simulink model "px4_allSensorsDemo"  (R2018b)
settings: Solver=FixedStepAuto  StartTime=0.0  StopTime=inf  RelTol=1e-3  EnableMultiTasking=on
libraries: px4Sensorslib x3, simulink_extras x3, px4uORBlib x2
settings Model: SimulationMode=external  ExtModeEnableFloating=off  ExtModeTrigDuration=10  Creator=The MathWorks, Inc.  LastModifiedBy=Tejas Rajopadhye
settings SolverCC: PositivePriorityOrder=on
settings DataIOCC: ReturnWorkspaceOutputs=on
settings OptimizationCC: EnhancedBackFolding=on  PassReuseOutputArgsAs=Individual arguments  MaxStackSize=64  OptimizeBlockOrder=speed  DifferentSizesBufferReuse=on  OptimizationCustomize=off
settings DebuggingCC: ParameterTunabilityLossMsg=error
settings HardwareCC: ProdBitPerPointer=32  ProdBitPerSizeT=32  ProdBitPerPtrDiffT=32  ProdLargestAtomicInteger=Long  ProdLargestAtomicFloat=Double  ProdWordSize=32  ProdLongLongMode=on  ProdHWDeviceType=ARM Compatible->ARM Cortex
settings SFSimCC: MATLABDynamicMemAlloc=off
settings RTWCC: SystemTargetFile=ert.tlc  HardwareBoard=PX4 Pixhawk 4  TLCOptions="-aInlineSetEventsForThisBaseRateFcn=TLC_FALSE -aSuppressMultiTaskScheduler=TLC_FALSE  -aRateBasedStepFcn=0"  TemplateMakefile=ert_default_tmf  GenerateReport=on  Toolchain=GNU Tools for PX4 Autopilots  IncludeHyperlinkInReport=on  LaunchReport=on  TargetLang=C++  GenerateTraceInfo=on  GenerateTraceReport=on  GenerateTraceReportSl=on  GenerateTraceReportSf=on  GenerateTraceReportEml=on
settings CodeAppCC: ForceParamTrailComments=on  IgnoreCustomStorageClasses=off  OperatorAnnotations=on  SimulinkDataObjDesc=on  SFDataObjDesc=on  InsertBlockDesc=on

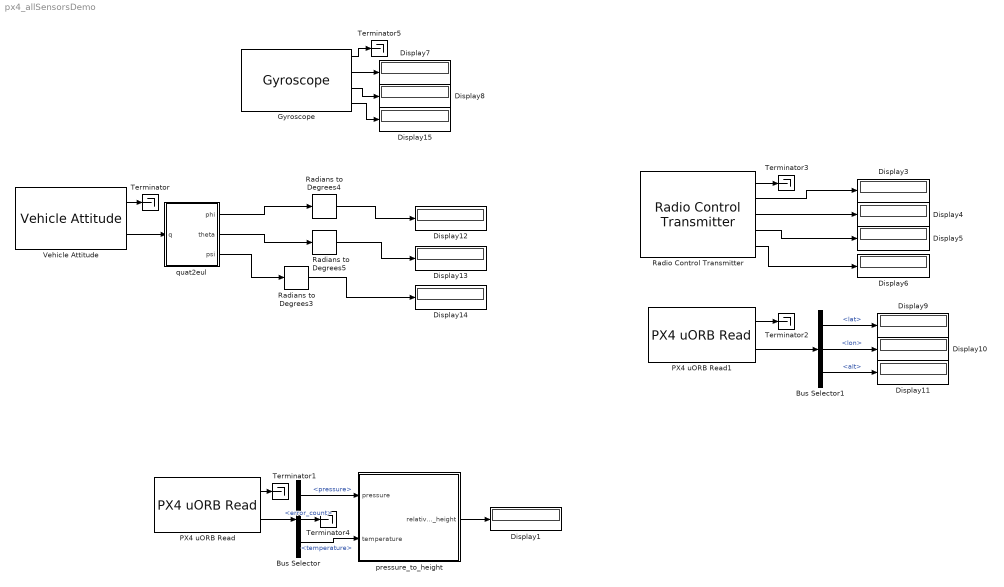
== system px4_allSensorsDemo ==
  Bus Selector : BusSelector  OutputSignals=pressure,error_count,temperature
  Bus Selector1 : BusSelector  OutputSignals=lat,lon,alt
  Display{1,3..15} (14 alike) : Display
  Gyroscope : px4Sensorslib/Gyroscope  uorbTimeStamp=off  BlockingMode=off  BlockTimeout=1e-3  sampleTime=1/250
      settings: SourceProductName=Embedded Coder Support Package for PX4 Autopilots
  PX4 uORB Read : px4uORBlib/PX4 uORB Read  uORBTopic=sensor_baro  sampleTime=-1  BlockingMode=off  BlockTimeout=1e-3
      settings: SourceProductName=Embedded Coder Support Package for PX4 Autopilots
  PX4 uORB Read1 : px4uORBlib/PX4 uORB Read  uORBTopic=vehicle_gps_position  sampleTime=-1  BlockingMode=off  BlockTimeout=1e-3
      settings: SourceProductName=Embedded Coder Support Package for PX4 Autopilots
  Radians to Degrees3 : simulink_extras/Transformations/Radians to Degrees
  Radians to Degrees4 : simulink_extras/Transformations/Radians to Degrees
  Radians to Degrees5 : simulink_extras/Transformations/Radians to Degrees
  Radio Control Transmitter : px4Sensorslib/Radio Control Transmitter  channel1=on  channel2=on  channel3=on  channel4=on  channel5=off  channel6=off  channel7=off  channel8=off  channel_count=off  rssi=off  rc_input_source=off  timestamp_last_signal=off  time_stamp=off  sampleTime=1/250  BlockingMode=off  BlockTimeout=5
      settings: SourceProductName=Embedded Coder Support Package for PX4 Autopilots
  Terminator{,1..5} (6 alike) : Terminator
  Vehicle Attitude : px4Sensorslib/Vehicle Attitude  rollRate=off  pitchRate=off  yawRate=off  quaternion=on  uorbTimeStamp=off  BlockingMode=off  BlockTimeout=0.001  sampleTime=1/250
      settings: SourceProductName=Embedded Coder Support Package for PX4 Autopilots
  pressure_to_height : MATLAB Function  TreatAsAtomicUnit=on
  quat2eul : MATLAB Function  TreatAsAtomicUnit=on
  wires:
  Vehicle Attitude/1 -> Terminator/1
  Vehicle Attitude/2 -> quat2eul/1(q)
  quat2eul/1(phi) -> Radians to Degrees4/1
  quat2eul/2(theta) -> Radians to Degrees5/1
  quat2eul/3(psi) -> Radians to Degrees3/1
  Radians to Degrees3/1 -> Display14/1
  Radians to Degrees4/1 -> Display12/1
  Radians to Degrees5/1 -> Display13/1
  PX4 uORB Read1/2 -> Bus Selector1/1
  PX4 uORB Read1/1 -> Terminator2/1
  Bus Selector1/1 -> Display9/1  "<lat>"
  Bus Selector1/2 -> Display10/1  "<lon>"
  Bus Selector1/3 -> Display11/1  "<alt>"
  Bus Selector/3 -> pressure_to_height/2(temperature)  "<temperature>"
  Bus Selector/1 -> pressure_to_height/1(pressure)  "<pressure>"
  PX4 uORB Read/1 -> Terminator1/1
  PX4 uORB Read/2 -> Bus Selector/1
  Bus Selector/2 -> Terminator4/1  "<error_count>"
  pressure_to_height/1(relative_height) -> Display1/1
  Radio Control Transmitter/2 -> Display3/1
  Radio Control Transmitter/3 -> Display4/1
  Radio Control Transmitter/4 -> Display5/1
  Radio Control Transmitter/5 -> Display6/1
  Radio Control Transmitter/1 -> Terminator3/1
  Gyroscope/2 -> Display7/1
  Gyroscope/3 -> Display8/1
  Gyroscope/4 -> Display15/1
  Gyroscope/1 -> Terminator5/1

== matlab function px4_allSensorsDemo/pressure_to_height ==
  data: pressure input; relative_height output; temperature input
function relative_height = covert_pressure_to_height(pressure, temperature)
R = single(287.058);
g = single(9.81);
temperature = temperature + single(273.15); %convert to kelvin from degrees

persistent itr;
if isempty(itr)
    itr = 0;
end

persistent init_pressure;
if isempty(init_pressure)
    init_pressure = single(944.77);
end

persistent initial_temp;
if isempty(initial_temp)
    initial_temp = temperature;
end

if (itr == 0)
    initial_pressure = pressure;
    itr = itr + 1;
else
    initial_pressure = single(init_pressure);
end

if (isreal(log(initial_pressure/pressure)))
    log_value = log(initial_pressure/pressure);
else
    log_value = 0;
end

init_pressure = single(initial_pressure);

relative_height = single(((R*initial_temp)/g)*log_value);

== matlab function px4_allSensorsDemo/quat2eul ==
  data: q input; phi output; theta output; psi output
function [phi,theta,psi] = quat2eul(q)

% Quaternion conversion to Euler angles based on the PX4 Firmware v1.6.5
% release.

phi = atan2(2*(q(1)*q(2) + q(3)* q(4)), q(1)^2 - q(2)^2 - q(3)^2 + q(4)^2);
theta = asin(-2*(q(2)*q(4) - q(1)*q(3)));
psi = atan2(2*(q(2)*q(3) + q(1)* q(4)), q(1)^2 + q(2)^2 - q(3)^2 - q(4)^2);

end
